simulink model "EPT"  (R2019b)
settings: Solver=FixedStepDiscrete  StartTime=0.0  StopTime=5  FixedStep=0.005  RelTol=1e-3  EnableMultiTasking=on
PreLoadFcn:
  | try, model_open; catch, disp('Error occurred while executing model pre-load callback: model_open.m'); disp('Please assure that the MATLAB working directory is set to the model directory before opening.'); end
InitFcn:
  | try, model_open; catch, end
undefined symbols (not defined in the file or in its folder): Bridge, GCM, H, ln, raptor_get_param_eval, raptor_get_safe_string, raptor_xcp_function
libraries: Raptor_lib x2810, simulink x374, hdlsllib x19
(part 35 of 45)

== system EPT/Foreground_TimeBase_5ms/E//W /BP-OBU_E//W/BP-OBU_E//W/BP-OBU_Warning//Fault_G3/BP-OBU_Warning_G3 ==
  Compare To Constant1 : simulink/Logic and Bit Operations/Compare To Constant  relop===  const=0  OutDataTypeStr=boolean
  Constant6 : Constant  Value=4
  Delay25 : Subsystem
  Delay26 : Subsystem
  Delay27 : Subsystem
  Delay28 : Subsystem
  Delay29 : Subsystem
  Latch26 : Subsystem
  Latch27 : Subsystem
  Latch28 : Subsystem
  Latch29 : Subsystem
  Logical Operator8 : Logic  Operator=OR  Inputs=7  AllPortsSameDT=off  OutDataTypeStr=boolean
  SOA : Subsystem
  raptor_adjustment82 : Raptor_lib/Data Storage/raptor_adjustment  paramName='Cdrive_Open'  nameSource=Parameter  initValue=0  dataType=boolean  storage=Calibration  calDispType=Number  calEnum={'False', 'True'}  calGain=1.0  calOffset=0.0  calMax=inf  calMin=-inf  calFormat='-1'  calUnit=''  calHelp=''  calAccess=1  calFunction=raptor_xcp_function(gcb)  calDispHeaders=off  calColHeaders={'Col1' 'Col2' 'Col3'}  calRowHeaders={'Row1' 'Row2' 'Row3'}
      settings: SourceProductName=Raptor
  raptor_adjustment83 : Raptor_lib/Data Storage/raptor_adjustment  paramName='Cchg_Open'  nameSource=Parameter  initValue=0  dataType=boolean  storage=Calibration  calDispType=Number  calEnum={'False', 'True'}  calGain=1.0  calOffset=0.0  calMax=inf  calMin=-inf  calFormat='-1'  calUnit=''  calHelp=''  calAccess=1  calFunction=raptor_xcp_function(gcb)  calDispHeaders=off  calColHeaders={'Col1' 'Col2' 'Col3'}  calRowHeaders={'Row1' 'Row2' 'Row3'}
      settings: SourceProductName=Raptor
  raptor_adjustment84 : Raptor_lib/Data Storage/raptor_adjustment  paramName='Caux_Open'  nameSource=Parameter  initValue=0  dataType=boolean  storage=Calibration  calDispType=Number  calEnum={'False', 'True'}  calGain=1.0  calOffset=0.0  calMax=inf  calMin=-inf  calFormat='-1'  calUnit=''  calHelp=''  calAccess=1  calFunction=raptor_xcp_function(gcb)  calDispHeaders=off  calColHeaders={'Col1' 'Col2' 'Col3'}  calRowHeaders={'Row1' 'Row2' 'Row3'}
      settings: SourceProductName=Raptor
  raptor_adjustment85 : Raptor_lib/Data Storage/raptor_adjustment  paramName='Csp_Open'  nameSource=Parameter  initValue=0  dataType=boolean  storage=Calibration  calDispType=Number  calEnum={'False', 'True'}  calGain=1.0  calOffset=0.0  calMax=inf  calMin=-inf  calFormat='-1'  calUnit=''  calHelp=''  calAccess=1  calFunction=raptor_xcp_function(gcb)  calDispHeaders=off  calColHeaders={'Col1' 'Col2' 'Col3'}  calRowHeaders={'Row1' 'Row2' 'Row3'}
      settings: SourceProductName=Raptor
  raptor_adjustment86 : Raptor_lib/Data Storage/raptor_adjustment  paramName='Fault_Cdrive_Open_1s_TimeCount'  nameSource=Parameter  initValue=200  dataType=double  storage=Calibration  calDispType=Number  calEnum={'False', 'True'}  calGain=1.0  calOffset=0.0  calMax=inf  calMin=-inf  calFormat='-1'  calUnit=''  calHelp=''  calAccess=1  calFunction=raptor_xcp_function(gcb)  calDispHeaders=off  calColHeaders={'Col1' 'Col2' 'Col3'}  calRowHeaders={'Row1' 'Row2' 'Row3'}
      settings: SourceProductName=Raptor
  raptor_adjustment87 : Raptor_lib/Data Storage/raptor_adjustment  paramName='Fault_Cchg_Open_1s_TimeCount'  nameSource=Parameter  initValue=200  dataType=double  storage=Calibration  calDispType=Number  calEnum={'False', 'True'}  calGain=1.0  calOffset=0.0  calMax=inf  calMin=-inf  calFormat='-1'  calUnit=''  calHelp=''  calAccess=1  calFunction=raptor_xcp_function(gcb)  calDispHeaders=off  calColHeaders={'Col1' 'Col2' 'Col3'}  calRowHeaders={'Row1' 'Row2' 'Row3'}
      settings: SourceProductName=Raptor
  raptor_adjustment88 : Raptor_lib/Data Storage/raptor_adjustment  paramName='Fault_Caux_Open_1s_TimeCount'  nameSource=Parameter  initValue=200  dataType=double  storage=Calibration  calDispType=Number  calEnum={'False', 'True'}  calGain=1.0  calOffset=0.0  calMax=inf  calMin=-inf  calFormat='-1'  calUnit=''  calHelp=''  calAccess=1  calFunction=raptor_xcp_function(gcb)  calDispHeaders=off  calColHeaders={'Col1' 'Col2' 'Col3'}  calRowHeaders={'Row1' 'Row2' 'Row3'}
      settings: SourceProductName=Raptor
  raptor_adjustment89 : Raptor_lib/Data Storage/raptor_adjustment  paramName='Fault_Csp_Open_1s_TimeCount'  nameSource=Parameter  initValue=200  dataType=double  storage=Calibration  calDispType=Number  calEnum={'False', 'True'}  calGain=1.0  calOffset=0.0  calMax=inf  calMin=-inf  calFormat='-1'  calUnit=''  calHelp=''  calAccess=1  calFunction=raptor_xcp_function(gcb)  calDispHeaders=off  calColHeaders={'Col1' 'Col2' 'Col3'}  calRowHeaders={'Row1' 'Row2' 'Row3'}
      settings: SourceProductName=Raptor
  raptor_data_def1 : Raptor_lib/Data Storage/raptor_data_def  dataName='Fault_SOA_OutOfRange'  initValue=0  dataType=boolean  storage=Calibration  calVisible=on  calType=Measurement  calDispType=Number  calEnum={'False', 'True'}  calGain=1.0  calOffset=0  calMin=-inf  calMax=inf  calFormat='-1'  calUnit=''  calHelp=''  calAccess=1  calFunction=raptor_xcp_function(gcb)  calDispHeaders=off  calColHeaders={'Col1' 'Col2' 'Col3'}  calRowHeaders={'Row1' 'Row2' 'Row3'}
      settings: SourceProductName=Raptor
  raptor_data_def10 : Raptor_lib/Data Storage/raptor_data_def  dataName='Warning_Cchg_Open'  initValue=0  dataType=boolean  storage=Calibration  calVisible=on  calType=Measurement  calDispType=Number  calEnum={'False', 'True'}  calGain=1.0  calOffset=0  calMin=-inf  calMax=inf  calFormat='-1'  calUnit=''  calHelp=''  calAccess=1  calFunction=raptor_xcp_function(gcb)  calDispHeaders=off  calColHeaders={'Col1' 'Col2' 'Col3'}  calRowHeaders={'Row1' 'Row2' 'Row3'}
      settings: SourceProductName=Raptor
  raptor_data_def11 : Raptor_lib/Data Storage/raptor_data_def  dataName='Warning_Caux_Open'  initValue=0  dataType=boolean  storage=Calibration  calVisible=on  calType=Measurement  calDispType=Number  calEnum={'False', 'True'}  calGain=1.0  calOffset=0  calMin=-inf  calMax=inf  calFormat='-1'  calUnit=''  calHelp=''  calAccess=1  calFunction=raptor_xcp_function(gcb)  calDispHeaders=off  calColHeaders={'Col1' 'Col2' 'Col3'}  calRowHeaders={'Row1' 'Row2' 'Row3'}
      settings: SourceProductName=Raptor
  raptor_data_def12 : Raptor_lib/Data Storage/raptor_data_def  dataName='Warning_Csp_Open'  initValue=0  dataType=boolean  storage=Calibration  calVisible=on  calType=Measurement  calDispType=Number  calEnum={'False', 'True'}  calGain=1.0  calOffset=0  calMin=-inf  calMax=inf  calFormat='-1'  calUnit=''  calHelp=''  calAccess=1  calFunction=raptor_xcp_function(gcb)  calDispHeaders=off  calColHeaders={'Col1' 'Col2' 'Col3'}  calRowHeaders={'Row1' 'Row2' 'Row3'}
      settings: SourceProductName=Raptor
  raptor_data_def2 : Raptor_lib/Data Storage/raptor_data_def  dataName='Warning_EndOfDischarge'  initValue=0  dataType=boolean  storage=Calibration  calVisible=on  calType=Measurement  calDispType=Number  calEnum={'False', 'True'}  calGain=1.0  calOffset=0  calMin=-inf  calMax=inf  calFormat='-1'  calUnit=''  calHelp=''  calAccess=1  calFunction=raptor_xcp_function(gcb)  calDispHeaders=off  calColHeaders={'Col1' 'Col2' 'Col3'}  calRowHeaders={'Row1' 'Row2' 'Row3'}
      settings: SourceProductName=Raptor
  raptor_data_def27 : Raptor_lib/Data Storage/raptor_data_def  dataName='Warning_EndOfCharge'  initValue=0  dataType=boolean  storage=Calibration  calVisible=on  calType=Measurement  calDispType=Number  calEnum={'False', 'True'}  calGain=1.0  calOffset=0  calMin=-inf  calMax=inf  calFormat='-1'  calUnit=''  calHelp=''  calAccess=1  calFunction=raptor_xcp_function(gcb)  calDispHeaders=off  calColHeaders={'Col1' 'Col2' 'Col3'}  calRowHeaders={'Row1' 'Row2' 'Row3'}
      settings: SourceProductName=Raptor
  raptor_data_def3 : Raptor_lib/Data Storage/raptor_data_def  dataName='Warning_SOA_OutOfRange'  initValue=0  dataType=boolean  storage=Calibration  calVisible=on  calType=Measurement  calDispType=Number  calEnum={'False', 'True'}  calGain=1.0  calOffset=0  calMin=-inf  calMax=inf  calFormat='-1'  calUnit=''  calHelp=''  calAccess=1  calFunction=raptor_xcp_function(gcb)  calDispHeaders=off  calColHeaders={'Col1' 'Col2' 'Col3'}  calRowHeaders={'Row1' 'Row2' 'Row3'}
      settings: SourceProductName=Raptor
  raptor_data_def4 : Raptor_lib/Data Storage/raptor_data_def  dataName='Fault_Cdrive_Open'  initValue=0  dataType=boolean  storage=Calibration  calVisible=on  calType=Measurement  calDispType=Number  calEnum={'False', 'True'}  calGain=1.0  calOffset=0  calMin=-inf  calMax=inf  calFormat='-1'  calUnit=''  calHelp=''  calAccess=1  calFunction=raptor_xcp_function(gcb)  calDispHeaders=off  calColHeaders={'Col1' 'Col2' 'Col3'}  calRowHeaders={'Row1' 'Row2' 'Row3'}
      settings: SourceProductName=Raptor
  raptor_data_def5 : Raptor_lib/Data Storage/raptor_data_def  dataName='Fault_Cchg_Open'  initValue=0  dataType=boolean  storage=Calibration  calVisible=on  calType=Measurement  calDispType=Number  calEnum={'False', 'True'}  calGain=1.0  calOffset=0  calMin=-inf  calMax=inf  calFormat='-1'  calUnit=''  calHelp=''  calAccess=1  calFunction=raptor_xcp_function(gcb)  calDispHeaders=off  calColHeaders={'Col1' 'Col2' 'Col3'}  calRowHeaders={'Row1' 'Row2' 'Row3'}
      settings: SourceProductName=Raptor
  raptor_data_def6 : Raptor_lib/Data Storage/raptor_data_def  dataName='Fault_Caux_Open'  initValue=0  dataType=boolean  storage=Calibration  calVisible=on  calType=Measurement  calDispType=Number  calEnum={'False', 'True'}  calGain=1.0  calOffset=0  calMin=-inf  calMax=inf  calFormat='-1'  calUnit=''  calHelp=''  calAccess=1  calFunction=raptor_xcp_function(gcb)  calDispHeaders=off  calColHeaders={'Col1' 'Col2' 'Col3'}  calRowHeaders={'Row1' 'Row2' 'Row3'}
      settings: SourceProductName=Raptor
  raptor_data_def7 : Raptor_lib/Data Storage/raptor_data_def  dataName='Fault_Csp_Open'  initValue=0  dataType=boolean  storage=Calibration  calVisible=on  calType=Measurement  calDispType=Number  calEnum={'False', 'True'}  calGain=1.0  calOffset=0  calMin=-inf  calMax=inf  calFormat='-1'  calUnit=''  calHelp=''  calAccess=1  calFunction=raptor_xcp_function(gcb)  calDispHeaders=off  calColHeaders={'Col1' 'Col2' 'Col3'}  calRowHeaders={'Row1' 'Row2' 'Row3'}
      settings: SourceProductName=Raptor
  raptor_data_def8 : Raptor_lib/Data Storage/raptor_data_def  dataName='HV_Off'  initValue=0  dataType=boolean  storage=Calibration  calVisible=on  calType=Measurement  calDispType=Number  calEnum={'False', 'True'}  calGain=1.0  calOffset=0  calMin=-inf  calMax=inf  calFormat='-1'  calUnit=''  calHelp=''  calAccess=1  calFunction=raptor_xcp_function(gcb)  calDispHeaders=off  calColHeaders={'Col1' 'Col2' 'Col3'}  calRowHeaders={'Row1' 'Row2' 'Row3'}
      settings: SourceProductName=Raptor
  raptor_data_def9 : Raptor_lib/Data Storage/raptor_data_def  dataName='Warning_Cdrive_Open'  initValue=0  dataType=boolean  storage=Calibration  calVisible=on  calType=Measurement  calDispType=Number  calEnum={'False', 'True'}  calGain=1.0  calOffset=0  calMin=-inf  calMax=inf  calFormat='-1'  calUnit=''  calHelp=''  calAccess=1  calFunction=raptor_xcp_function(gcb)  calDispHeaders=off  calColHeaders={'Col1' 'Col2' 'Col3'}  calRowHeaders={'Row1' 'Row2' 'Row3'}
      settings: SourceProductName=Raptor
  raptor_data_read : Raptor_lib/Data Storage/raptor_data_read  dataName='Warning_EndOfCharge'  dataShape=Scalar  idxSource=Input  idxRow=1  idxCol=1
      settings: SourceProductName=Raptor
  raptor_data_read1 : Raptor_lib/Data Storage/raptor_data_read  dataName='Warning_EndOfDischarge'  dataShape=Scalar  idxSource=Input  idxRow=1  idxCol=1
      settings: SourceProductName=Raptor
  raptor_data_read14 : Raptor_lib/Data Storage/raptor_data_read  dataName='Fault_Reset_Trigger'  dataShape=Scalar  idxSource=Input  idxRow=1  idxCol=1
      settings: SourceProductName=Raptor
  raptor_data_read3 : Raptor_lib/Data Storage/raptor_data_read  dataName='CMU_Ready'  dataShape=Scalar  idxSource=Input  idxRow=1  idxCol=1
      settings: SourceProductName=Raptor
  raptor_data_write10 : Raptor_lib/Data Storage/raptor_data_write  dataName='Warning_Cchg_Open'  dataShape=Scalar  idxSource=Input Port  idxRow=1  idxCol=1
      settings: SourceProductName=Raptor
  raptor_data_write11 : Raptor_lib/Data Storage/raptor_data_write  dataName='Warning_Csp_Open'  dataShape=Scalar  idxSource=Input Port  idxRow=1  idxCol=1
      settings: SourceProductName=Raptor
  raptor_data_write3 : Raptor_lib/Data Storage/raptor_data_write  dataName='Fault_Caux_Open'  dataShape=Scalar  idxSource=Input Port  idxRow=1  idxCol=1
      settings: SourceProductName=Raptor
  raptor_data_write4 : Raptor_lib/Data Storage/raptor_data_write  dataName='Fault_Cdrive_Open'  dataShape=Scalar  idxSource=Input Port  idxRow=1  idxCol=1
      settings: SourceProductName=Raptor
  raptor_data_write5 : Raptor_lib/Data Storage/raptor_data_write  dataName='Fault_Cchg_Open'  dataShape=Scalar  idxSource=Input Port  idxRow=1  idxCol=1
      settings: SourceProductName=Raptor
  raptor_data_write6 : Raptor_lib/Data Storage/raptor_data_write  dataName='Fault_Csp_Open'  dataShape=Scalar  idxSource=Input Port  idxRow=1  idxCol=1
      settings: SourceProductName=Raptor
  raptor_data_write7 : Raptor_lib/Data Storage/raptor_data_write  dataName='HV_Off'  dataShape=Scalar  idxSource=Input Port  idxRow=1  idxCol=1
      settings: SourceProductName=Raptor
  raptor_data_write8 : Raptor_lib/Data Storage/raptor_data_write  dataName='Warning_Caux_Open'  dataShape=Scalar  idxSource=Input Port  idxRow=1  idxCol=1
      settings: SourceProductName=Raptor
  raptor_data_write9 : Raptor_lib/Data Storage/raptor_data_write  dataName='Warning_Cdrive_Open'  dataShape=Scalar  idxSource=Input Port  idxRow=1  idxCol=1
      settings: SourceProductName=Raptor
  raptor_override : Raptor_lib/Data Storage/raptor_override  paramName='Cal_HV_Off'  nameSource=Parameter  measurement=None  calDispType=Number  calEnum={'False', 'True'}  calGain=1.0  calOffset=0.0  calMax=inf  calMin=-inf  calFormat='-1'  calUnit=''  calHelp=''  calAccess=1  calFunction=[raptor_xcp_function(gcb) '|' raptor_get_param_eval(gcb, 'paramName') '_Override']
      settings: SourceProductName=Raptor
  Warning_SOA_OutOfRange : Outport  VectorParamsAs1DForOutWhenUnconnected=off
  Warning_CMU_Status : Outport  Port=2  VectorParamsAs1DForOutWhenUnconnected=off
  Warning_Cdrive_Open : Outport  Port=3  VectorParamsAs1DForOutWhenUnconnected=off
  Warning_Cchg_Open : Outport  Port=4  VectorParamsAs1DForOutWhenUnconnected=off
  Warning_Caux_Open : Outport  Port=5  VectorParamsAs1DForOutWhenUnconnected=off
  Warning_Csp_Open : Outport  Port=6  VectorParamsAs1DForOutWhenUnconnected=off
  Fault_Cdrive_Open : Outport  Port=7  VectorParamsAs1DForOutWhenUnconnected=off
  Fault_Cchg_Open : Outport  Port=8  VectorParamsAs1DForOutWhenUnconnected=off
  Warning_Cdrive_Open3 : Outport  Port=9  VectorParamsAs1DForOutWhenUnconnected=off
  Fault_Csp_Open : Outport  Port=10  VectorParamsAs1DForOutWhenUnconnected=off
  wires:
  Latch28/1(Output) -> Warning_Cdrive_Open3/1, raptor_data_write3/1
  Delay27/1(Output) -> Latch27/1(Latch)
  Compare To Constant1/1 -> Delay25/1(Condition), Warning_CMU_Status/1
  raptor_adjustment82/1 -> Delay26/1(Condition), Logical Operator8/4, Warning_Cdrive_Open/1, raptor_data_write9/1
  raptor_data_read3/1 -> Compare To Constant1/1
  raptor_adjustment86/1 -> Delay26/2(TimeCount)
  Latch27/1(Output) -> Fault_Cchg_Open/1, raptor_data_write5/1
  Delay26/1(Output) -> Latch26/1(Latch)
  raptor_adjustment84/1 -> Delay28/1(Condition), Logical Operator8/6, Warning_Caux_Open/1, raptor_data_write8/1
  Logical Operator8/1 -> raptor_override/1
  raptor_adjustment89/1 -> Delay29/2(TimeCount)
  Latch29/1(Output) -> Fault_Csp_Open/1, raptor_data_write6/1
  raptor_adjustment85/1 -> Delay29/1(Condition), Logical Operator8/7, raptor_data_write11/1, Warning_Csp_Open/1
  raptor_adjustment87/1 -> Delay27/2(TimeCount)
  Latch26/1(Output) -> Fault_Cdrive_Open/1, raptor_data_write4/1
  Delay25/1(Output) -> Logical Operator8/3
  Constant6/1 -> Delay25/2(TimeCount)
  Delay29/1(Output) -> Latch29/1(Latch)
  Delay28/1(Output) -> Latch28/1(Latch)
  raptor_adjustment88/1 -> Delay28/2(TimeCount)
  raptor_adjustment83/1 -> Delay27/1(Condition), Logical Operator8/5, raptor_data_write10/1, Warning_Cchg_Open/1
  raptor_data_read14/1 -> Latch26/2(Reset), Latch27/2(Reset), Latch28/2(Reset), Latch29/2(Reset)
  raptor_data_read/1 -> Logical Operator8/1
  raptor_data_read1/1 -> Logical Operator8/2
  SOA/1(Out1) -> Warning_SOA_OutOfRange/1
  raptor_override/1 -> raptor_data_write7/1

== system EPT/Foreground_TimeBase_5ms/E//W /BP-OBU_E//W/BP-OBU_E//W/BP-OBU_Warning//Fault_G5/BP-OBU_Fault_G5 ==
  "MCU Work " : Inport
  Delay : Subsystem
  Delay1 : Subsystem
  Delay2 : Subsystem
  Delay3 : Subsystem
  Delay4 : Subsystem
  Delay5 : Subsystem
  Delay6 : Subsystem
  Error : Subsystem
  Error1 : Subsystem
  Error2 : Subsystem
  Error3 : Subsystem
  Error5 : Subsystem
  Error6 : Subsystem
  Error7 : Subsystem
  Logical Operator11 : Logic  AllPortsSameDT=off  OutDataTypeStr=boolean
  Logical Operator12 : Logic  AllPortsSameDT=off  OutDataTypeStr=boolean
  Logical Operator13 : Logic  AllPortsSameDT=off  OutDataTypeStr=boolean
  Relational Operator10 : RelationalOperator  Operator=<=  OutDataTypeStr=boolean  RndMeth=Simplest
  Relational Operator{7,9,12..14} (5 alike) : RelationalOperator  OutDataTypeStr=boolean  RndMeth=Simplest
  Relational Operator8 : RelationalOperator  Operator=<=  OutDataTypeStr=boolean  RndMeth=Simplest
  raptor_adjustment10 : Raptor_lib/Data Storage/raptor_adjustment  paramName='Fault__Sensor_Voltage_LowerLimit'  nameSource=Parameter  initValue=4  dataType=double  storage=Calibration  calDispType=Number  calEnum={'False', 'True'}  calGain=1.0  calOffset=0.0  calMax=inf  calMin=-inf  calFormat='-1'  calUnit=''  calHelp=''  calAccess=1  calFunction=raptor_xcp_function(gcb)  calDispHeaders=off  calColHeaders={'Col1' 'Col2' 'Col3'}  calRowHeaders={'Row1' 'Row2' 'Row3'}
      settings: SourceProductName=Raptor
  raptor_adjustment11 : Raptor_lib/Data Storage/raptor_adjustment  paramName='Fault_Sensor_Voltage_TimeCount'  nameSource=Parameter  initValue=20  dataType=double  storage=Calibration  calDispType=Number  calEnum={'False', 'True'}  calGain=1.0  calOffset=0.0  calMax=inf  calMin=-inf  calFormat='-1'  calUnit=''  calHelp=''  calAccess=1  calFunction=raptor_xcp_function(gcb)  calDispHeaders=off  calColHeaders={'Col1' 'Col2' 'Col3'}  calRowHeaders={'Row1' 'Row2' 'Row3'}
      settings: SourceProductName=Raptor
  raptor_adjustment12 : Raptor_lib/Data Storage/raptor_adjustment  paramName='Fault_Temperature_MCU_UpperLimit'  nameSource=Parameter  initValue=85  dataType=double  storage=Calibration  calDispType=Number  calEnum={'False', 'True'}  calGain=1.0  calOffset=0.0  calMax=inf  calMin=-inf  calFormat='-1'  calUnit=''  calHelp=''  calAccess=1  calFunction=raptor_xcp_function(gcb)  calDispHeaders=off  calColHeaders={'Col1' 'Col2' 'Col3'}  calRowHeaders={'Row1' 'Row2' 'Row3'}
      settings: SourceProductName=Raptor
  raptor_adjustment13 : Raptor_lib/Data Storage/raptor_adjustment  paramName='Fault_Temperature_Motor_UpperLimit'  nameSource=Parameter  initValue=135  dataType=double  storage=Calibration  calDispType=Number  calEnum={'False', 'True'}  calGain=1.0  calOffset=0.0  calMax=inf  calMin=-inf  calFormat='-1'  calUnit=''  calHelp=''  calAccess=1  calFunction=raptor_xcp_function(gcb)  calDispHeaders=off  calColHeaders={'Col1' 'Col2' 'Col3'}  calRowHeaders={'Row1' 'Row2' 'Row3'}
      settings: SourceProductName=Raptor
  raptor_adjustment14 : Raptor_lib/Data Storage/raptor_adjustment  paramName='Fault_Motor_RPM_UpperLimit'  nameSource=Parameter  initValue=6500  dataType=double  storage=Calibration  calDispType=Number  calEnum={'False', 'True'}  calGain=1.0  calOffset=0.0  calMax=inf  calMin=-inf  calFormat='-1'  calUnit=''  calHelp=''  calAccess=1  calFunction=raptor_xcp_function(gcb)  calDispHeaders=off  calColHeaders={'Col1' 'Col2' 'Col3'}  calRowHeaders={'Row1' 'Row2' 'Row3'}
      settings: SourceProductName=Raptor
  raptor_adjustment15 : Raptor_lib/Data Storage/raptor_adjustment  paramName='Fault_Motor_RPM_TimeCount'  nameSource=Parameter  initValue=20  dataType=double  storage=Calibration  calDispType=Number  calEnum={'False', 'True'}  calGain=1.0  calOffset=0.0  calMax=inf  calMin=-inf  calFormat='-1'  calUnit=''  calHelp=''  calAccess=1  calFunction=raptor_xcp_function(gcb)  calDispHeaders=off  calColHeaders={'Col1' 'Col2' 'Col3'}  calRowHeaders={'Row1' 'Row2' 'Row3'}
      settings: SourceProductName=Raptor
  raptor_adjustment16 : Raptor_lib/Data Storage/raptor_adjustment  paramName='Fault_Temperature_Motor_TimeCount'  nameSource=Parameter  initValue=20  dataType=double  storage=Calibration  calDispType=Number  calEnum={'False', 'True'}  calGain=1.0  calOffset=0.0  calMax=inf  calMin=-inf  calFormat='-1'  calUnit=''  calHelp=''  calAccess=1  calFunction=raptor_xcp_function(gcb)  calDispHeaders=off  calColHeaders={'Col1' 'Col2' 'Col3'}  calRowHeaders={'Row1' 'Row2' 'Row3'}
      settings: SourceProductName=Raptor
  raptor_adjustment17 : Raptor_lib/Data Storage/raptor_adjustment  paramName='Fault_Temperature_MCU_TimeCount'  nameSource=Parameter  initValue=20  dataType=double  storage=Calibration  calDispType=Number  calEnum={'False', 'True'}  calGain=1.0  calOffset=0.0  calMax=inf  calMin=-inf  calFormat='-1'  calUnit=''  calHelp=''  calAccess=1  calFunction=raptor_xcp_function(gcb)  calDispHeaders=off  calColHeaders={'Col1' 'Col2' 'Col3'}  calRowHeaders={'Row1' 'Row2' 'Row3'}
      settings: SourceProductName=Raptor
  raptor_adjustment4 : Raptor_lib/Data Storage/raptor_adjustment  paramName='Fault_12VBattery_Voltage_TimeCount'  nameSource=Parameter  initValue=20  dataType=double  storage=Calibration  calDispType=Number  calEnum={'False', 'True'}  calGain=1.0  calOffset=0.0  calMax=inf  calMin=-inf  calFormat='-1'  calUnit=''  calHelp=''  calAccess=1  calFunction=raptor_xcp_function(gcb)  calDispHeaders=off  calColHeaders={'Col1' 'Col2' 'Col3'}  calRowHeaders={'Row1' 'Row2' 'Row3'}
      settings: SourceProductName=Raptor
  raptor_adjustment7 : Raptor_lib/Data Storage/raptor_adjustment  paramName='Fault_Battery_Voltage_UpperLimit'  nameSource=Parameter  initValue=15  dataType=double  storage=Calibration  calDispType=Number  calEnum={'False', 'True'}  calGain=1.0  calOffset=0.0  calMax=inf  calMin=-inf  calFormat='-1'  calUnit=''  calHelp=''  calAccess=1  calFunction=raptor_xcp_function(gcb)  calDispHeaders=off  calColHeaders={'Col1' 'Col2' 'Col3'}  calRowHeaders={'Row1' 'Row2' 'Row3'}
      settings: SourceProductName=Raptor
  raptor_adjustment8 : Raptor_lib/Data Storage/raptor_adjustment  paramName='Fault__Battery_Voltage_LowerLimit'  nameSource=Parameter  initValue=10  dataType=double  storage=Calibration  calDispType=Number  calEnum={'False', 'True'}  calGain=1.0  calOffset=0.0  calMax=inf  calMin=-inf  calFormat='-1'  calUnit=''  calHelp=''  calAccess=1  calFunction=raptor_xcp_function(gcb)  calDispHeaders=off  calColHeaders={'Col1' 'Col2' 'Col3'}  calRowHeaders={'Row1' 'Row2' 'Row3'}
      settings: SourceProductName=Raptor
  raptor_adjustment9 : Raptor_lib/Data Storage/raptor_adjustment  paramName='Fault_Sensor_Voltage_UpperLimit'  nameSource=Parameter  initValue=6  dataType=double  storage=Calibration  calDispType=Number  calEnum={'False', 'True'}  calGain=1.0  calOffset=0.0  calMax=inf  calMin=-inf  calFormat='-1'  calUnit=''  calHelp=''  calAccess=1  calFunction=raptor_xcp_function(gcb)  calDispHeaders=off  calColHeaders={'Col1' 'Col2' 'Col3'}  calRowHeaders={'Row1' 'Row2' 'Row3'}
      settings: SourceProductName=Raptor
  raptor_data_def11 : Raptor_lib/Data Storage/raptor_data_def  dataName='Fault_12V_Battery_Voltage_Low'  initValue=0  dataType=boolean  storage=Volatile (RAM)  calVisible=on  calType=Measurement  calDispType=Number  calEnum={'False', 'True'}  calGain=1.0  calOffset=0  calMin=-inf  calMax=inf  calFormat='-1'  calUnit=''  calHelp=''  calAccess=1  calFunction=raptor_xcp_function(gcb)  calDispHeaders=off  calColHeaders={'Col1' 'Col2' 'Col3'}  calRowHeaders={'Row1' 'Row2' 'Row3'}
      settings: SourceProductName=Raptor
  raptor_data_def12 : Raptor_lib/Data Storage/raptor_data_def  dataName='Fault_Sensor_Voltage_High'  initValue=0  dataType=boolean  storage=Volatile (RAM)  calVisible=on  calType=Measurement  calDispType=Number  calEnum={'False', 'True'}  calGain=1.0  calOffset=0  calMin=-inf  calMax=inf  calFormat='-1'  calUnit=''  calHelp=''  calAccess=1  calFunction=raptor_xcp_function(gcb)  calDispHeaders=off  calColHeaders={'Col1' 'Col2' 'Col3'}  calRowHeaders={'Row1' 'Row2' 'Row3'}
      settings: SourceProductName=Raptor
  raptor_data_def13 : Raptor_lib/Data Storage/raptor_data_def  dataName='Fault_Sensor_Voltage_Low'  initValue=0  dataType=boolean  storage=Volatile (RAM)  calVisible=on  calType=Measurement  calDispType=Number  calEnum={'False', 'True'}  calGain=1.0  calOffset=0  calMin=-inf  calMax=inf  calFormat='-1'  calUnit=''  calHelp=''  calAccess=1  calFunction=raptor_xcp_function(gcb)  calDispHeaders=off  calColHeaders={'Col1' 'Col2' 'Col3'}  calRowHeaders={'Row1' 'Row2' 'Row3'}
      settings: SourceProductName=Raptor
  raptor_data_def15 : Raptor_lib/Data Storage/raptor_data_def  dataName='Fault_Temperature_MCU_High'  initValue=0  dataType=boolean  storage=Volatile (RAM)  calVisible=on  calType=Measurement  calDispType=Number  calEnum={'False', 'True'}  calGain=1.0  calOffset=0  calMin=-inf  calMax=inf  calFormat='-1'  calUnit=''  calHelp=''  calAccess=1  calFunction=raptor_xcp_function(gcb)  calDispHeaders=off  calColHeaders={'Col1' 'Col2' 'Col3'}  calRowHeaders={'Row1' 'Row2' 'Row3'}
      settings: SourceProductName=Raptor
  raptor_data_def16 : Raptor_lib/Data Storage/raptor_data_def  dataName='Fault_Temperature_Motor_High'  initValue=0  dataType=boolean  storage=Volatile (RAM)  calVisible=on  calType=Measurement  calDispType=Number  calEnum={'False', 'True'}  calGain=1.0  calOffset=0  calMin=-inf  calMax=inf  calFormat='-1'  calUnit=''  calHelp=''  calAccess=1  calFunction=raptor_xcp_function(gcb)  calDispHeaders=off  calColHeaders={'Col1' 'Col2' 'Col3'}  calRowHeaders={'Row1' 'Row2' 'Row3'}
      settings: SourceProductName=Raptor
  raptor_data_def18 : Raptor_lib/Data Storage/raptor_data_def  dataName='Fault_Motor_RPM_High'  initValue=0  dataType=boolean  storage=Volatile (RAM)  calVisible=on  calType=Measurement  calDispType=Number  calEnum={'False', 'True'}  calGain=1.0  calOffset=0  calMin=-inf  calMax=inf  calFormat='-1'  calUnit=''  calHelp=''  calAccess=1  calFunction=raptor_xcp_function(gcb)  calDispHeaders=off  calColHeaders={'Col1' 'Col2' 'Col3'}  calRowHeaders={'Row1' 'Row2' 'Row3'}
      settings: SourceProductName=Raptor
  raptor_data_def9 : Raptor_lib/Data Storage/raptor_data_def  dataName='Fault_12V_Battery_Voltage_High'  initValue=0  dataType=boolean  storage=Volatile (RAM)  calVisible=on  calType=Measurement  calDispType=Number  calEnum={'False', 'True'}  calGain=1.0  calOffset=0  calMin=-inf  calMax=inf  calFormat='-1'  calUnit=''  calHelp=''  calAccess=1  calFunction=raptor_xcp_function(gcb)  calDispHeaders=off  calColHeaders={'Col1' 'Col2' 'Col3'}  calRowHeaders={'Row1' 'Row2' 'Row3'}
      settings: SourceProductName=Raptor
  raptor_data_read13 : Raptor_lib/Data Storage/raptor_data_read  dataName='Sensor_5V_Volt'  dataShape=Scalar  idxSource=Input  idxRow=1  idxCol=1
      settings: SourceProductName=Raptor
  raptor_data_read14 : Raptor_lib/Data Storage/raptor_data_read  dataName='Fault_Reset_Trigger'  dataShape=Scalar  idxSource=Input  idxRow=1  idxCol=1
      settings: SourceProductName=Raptor
  raptor_data_read4 : Raptor_lib/Data Storage/raptor_data_read  dataName='Read_Controller_Temp'  dataShape=Scalar  idxSource=Input  idxRow=1  idxCol=1
      settings: SourceProductName=Raptor
  raptor_data_read5 : Raptor_lib/Data Storage/raptor_data_read  dataName='Read_Motor_Temp'  dataShape=Scalar  idxSource=Input  idxRow=1  idxCol=1
      settings: SourceProductName=Raptor
  raptor_data_read6 : Raptor_lib/Data Storage/raptor_data_read  dataName='Read_Motor_Speed'  dataShape=Scalar  idxSource=Input  idxRow=1  idxCol=1
      settings: SourceProductName=Raptor
  raptor_data_read7 : Raptor_lib/Data Storage/raptor_data_read  dataName='I2V_Battery_Volt'  dataShape=Scalar  idxSource=Input  idxRow=1  idxCol=1
      settings: SourceProductName=Raptor
  raptor_data_write10 : Raptor_lib/Data Storage/raptor_data_write  dataName='Fault_Sensor_Voltage_High'  dataShape=Scalar  idxSource=Input Port  idxRow=1  idxCol=1
      settings: SourceProductName=Raptor
  raptor_data_write11 : Raptor_lib/Data Storage/raptor_data_write  dataName='Fault_12V_Battery_Voltage_High'  dataShape=Scalar  idxSource=Input Port  idxRow=1  idxCol=1
      settings: SourceProductName=Raptor
  raptor_data_write12 : Raptor_lib/Data Storage/raptor_data_write  dataName='Fault_12V_Battery_Voltage_Low'  dataShape=Scalar  idxSource=Input Port  idxRow=1  idxCol=1
      settings: SourceProductName=Raptor
  raptor_data_write13 : Raptor_lib/Data Storage/raptor_data_write  dataName='Fault_Sensor_Voltage_Low'  dataShape=Scalar  idxSource=Input Port  idxRow=1  idxCol=1
      settings: SourceProductName=Raptor
  raptor_data_write15 : Raptor_lib/Data Storage/raptor_data_write  dataName='Fault_Temperature_MCU_High'  dataShape=Scalar  idxSource=Input Port  idxRow=1  idxCol=1
      settings: SourceProductName=Raptor
  raptor_data_write16 : Raptor_lib/Data Storage/raptor_data_write  dataName='Fault_Temperature_Motor_High'  dataShape=Scalar  idxSource=Input Port  idxRow=1  idxCol=1
      settings: SourceProductName=Raptor
  raptor_data_write18 : Raptor_lib/Data Storage/raptor_data_write  dataName='Fault_Motor_RPM_High'  dataShape=Scalar  idxSource=Input Port  idxRow=1  idxCol=1
      settings: SourceProductName=Raptor
  wires:
  Delay2/1(Output) -> Error2/1(" Condition")
  raptor_data_read13/1 -> Relational Operator10/1, Relational Operator9/1
  raptor_adjustment15/1 -> Delay6/2(TimeCount)
  raptor_data_read14/1 -> Error7/2(" Reset"), Error6/2(" Reset"), Error5/2(" Reset"), Error3/2(" Reset"), Error2/2(" Reset"), Error1/2(" Reset"), Error/2(" Reset")
  raptor_data_read7/1 -> Relational Operator7/1, Relational Operator8/1
  "MCU Work "/1 -> Logical Operator13/1, Logical Operator12/1, Logical Operator11/1
  Logical Operator12/1 -> Delay5/1(Condition)
  Logical Operator11/1 -> Delay4/1(Condition)
  raptor_adjustment17/1 -> Delay4/2(TimeCount)
  Relational Operator9/1 -> Delay2/1(Condition)
  Relational Operator13/1 -> Logical Operator12/2
  Relational Operator10/1 -> Delay3/1(Condition)
  Error5/1(Error) -> raptor_data_write15/1
  raptor_adjustment4/1 -> Delay1/2(TimeCount), Delay/2(TimeCount)
  raptor_adjustment10/1 -> Relational Operator10/2
  raptor_adjustment12/1 -> Relational Operator12/2
  raptor_data_read4/1 -> Relational Operator12/1
  raptor_adjustment7/1 -> Relational Operator7/2
  Delay/1(Output) -> Error/1(" Condition")
  raptor_data_read5/1 -> Relational Operator13/1
  raptor_adjustment8/1 -> Relational Operator8/2
  raptor_adjustment14/1 -> Relational Operator14/2
  Error2/1(Error) -> raptor_data_write10/1
  raptor_adjustment9/1 -> Relational Operator9/2
  raptor_adjustment13/1 -> Relational Operator13/2
  Error1/1(Error) -> raptor_data_write12/1
  Relational Operator14/1 -> Logical Operator13/2
  Error3/1(Error) -> raptor_data_write13/1
  raptor_adjustment11/1 -> Delay2/2(TimeCount), Delay3/2(TimeCount)
  Relational Operator12/1 -> Logical Operator11/2
  Relational Operator7/1 -> Delay/1(Condition)
  Relational Operator8/1 -> Delay1/1(Condition)
  Logical Operator13/1 -> Delay6/1(Condition)
  Delay6/1(Output) -> Error7/1(" Condition")
  Delay3/1(Output) -> Error3/1(" Condition")
  raptor_adjustment16/1 -> Delay5/2(TimeCount)
  Delay1/1(Output) -> Error1/1(" Condition")
  Delay4/1(Output) -> Error5/1(" Condition")
  Delay5/1(Output) -> Error6/1(" Condition")
  Error/1(Error) -> raptor_data_write11/1
  raptor_data_read6/1 -> Relational Operator14/1
  Error7/1(Error) -> raptor_data_write18/1
  Error6/1(Error) -> raptor_data_write16/1

== system EPT/Foreground_TimeBase_5ms/E//W /BP-OBU_E//W/BP-OBU_E//W/BP-OBU_Warning//Fault_G5/BP-OBU_Warning_G5 ==
  "MCU Work " : Inport
  Logical Operator8 : Logic  AllPortsSameDT=off  OutDataTypeStr=boolean
  Logical Operator9 : Logic  AllPortsSameDT=off  OutDataTypeStr=boolean
  Relational Operator{,2,5..6} (4 alike) : RelationalOperator  OutDataTypeStr=boolean  RndMeth=Simplest
  Relational Operator1 : RelationalOperator  Operator=<=  OutDataTypeStr=boolean  RndMeth=Simplest
  Relational Operator3 : RelationalOperator  Operator=<=  OutDataTypeStr=boolean  RndMeth=Simplest
  raptor_adjustment : Raptor_lib/Data Storage/raptor_adjustment  paramName='Warning_12VBattery_Voltage_UpperLimit'  nameSource=Parameter  initValue=13.8  dataType=double  storage=Calibration  calDispType=Number  calEnum={'False', 'True'}  calGain=1.0  calOffset=0.0  calMax=inf  calMin=-inf  calFormat='-1'  calUnit=''  calHelp=''  calAccess=1  calFunction=raptor_xcp_function(gcb)  calDispHeaders=off  calColHeaders={'Col1' 'Col2' 'Col3'}  calRowHeaders={'Row1' 'Row2' 'Row3'}
      settings: SourceProductName=Raptor
  raptor_adjustment1 : Raptor_lib/Data Storage/raptor_adjustment  paramName='Warning_12VBattery_Voltage_LowerLimit'  nameSource=Parameter  initValue=11  dataType=double  storage=Calibration  calDispType=Number  calEnum={'False', 'True'}  calGain=1.0  calOffset=0.0  calMax=inf  calMin=-inf  calFormat='-1'  calUnit=''  calHelp=''  calAccess=1  calFunction=raptor_xcp_function(gcb)  calDispHeaders=off  calColHeaders={'Col1' 'Col2' 'Col3'}  calRowHeaders={'Row1' 'Row2' 'Row3'}
      settings: SourceProductName=Raptor
  raptor_adjustment2 : Raptor_lib/Data Storage/raptor_adjustment  paramName='Warning_Sensor_Voltage_UpperLimit'  nameSource=Parameter  initValue=5.5  dataType=double  storage=Calibration  calDispType=Number  calEnum={'False', 'True'}  calGain=1.0  calOffset=0.0  calMax=inf  calMin=-inf  calFormat='-1'  calUnit=''  calHelp=''  calAccess=1  calFunction=raptor_xcp_function(gcb)  calDispHeaders=off  calColHeaders={'Col1' 'Col2' 'Col3'}  calRowHeaders={'Row1' 'Row2' 'Row3'}
      settings: SourceProductName=Raptor
  raptor_adjustment3 : Raptor_lib/Data Storage/raptor_adjustment  paramName='Warning_Sensor_Voltage_LowerLimit'  nameSource=Parameter  initValue=4.5  dataType=double  storage=Calibration  calDispType=Number  calEnum={'False', 'True'}  calGain=1.0  calOffset=0.0  calMax=inf  calMin=-inf  calFormat='-1'  calUnit=''  calHelp=''  calAccess=1  calFunction=raptor_xcp_function(gcb)  calDispHeaders=off  calColHeaders={'Col1' 'Col2' 'Col3'}  calRowHeaders={'Row1' 'Row2' 'Row3'}
      settings: SourceProductName=Raptor
  raptor_adjustment5 : Raptor_lib/Data Storage/raptor_adjustment  paramName='Warning_Temperature_MCU_UpperLimit'  nameSource=Parameter  initValue=70  dataType=double  storage=Calibration  calDispType=Number  calEnum={'False', 'True'}  calGain=1.0  calOffset=0.0  calMax=inf  calMin=-inf  calFormat='-1'  calUnit=''  calHelp=''  calAccess=1  calFunction=raptor_xcp_function(gcb)  calDispHeaders=off  calColHeaders={'Col1' 'Col2' 'Col3'}  calRowHeaders={'Row1' 'Row2' 'Row3'}
      settings: SourceProductName=Raptor
  raptor_adjustment6 : Raptor_lib/Data Storage/raptor_adjustment  paramName='Warning_Temperature_Motor_UpperLimit'  nameSource=Parameter  initValue=100  dataType=double  storage=Calibration  calDispType=Number  calEnum={'False', 'True'}  calGain=1.0  calOffset=0.0  calMax=inf  calMin=-inf  calFormat='-1'  calUnit=''  calHelp=''  calAccess=1  calFunction=raptor_xcp_function(gcb)  calDispHeaders=off  calColHeaders={'Col1' 'Col2' 'Col3'}  calRowHeaders={'Row1' 'Row2' 'Row3'}
      settings: SourceProductName=Raptor
  raptor_data_def2 : Raptor_lib/Data Storage/raptor_data_def  dataName='Warning_12V_Battery_Voltage_High'  initValue=0  dataType=boolean  storage=Volatile (RAM)  calVisible=on  calType=Measurement  calDispType=Number  calEnum={'False', 'True'}  calGain=1.0  calOffset=0  calMin=-inf  calMax=inf  calFormat='-1'  calUnit=''  calHelp=''  calAccess=1  calFunction=raptor_xcp_function(gcb)  calDispHeaders=off  calColHeaders={'Col1' 'Col2' 'Col3'}  calRowHeaders={'Row1' 'Row2' 'Row3'}
      settings: SourceProductName=Raptor
  raptor_data_def3 : Raptor_lib/Data Storage/raptor_data_def  dataName='Warning_12V_Battery_Voltage_Low'  initValue=0  dataType=boolean  storage=Volatile (RAM)  calVisible=on  calType=Measurement  calDispType=Number  calEnum={'False', 'True'}  calGain=1.0  calOffset=0  calMin=-inf  calMax=inf  calFormat='-1'  calUnit=''  calHelp=''  calAccess=1  calFunction=raptor_xcp_function(gcb)  calDispHeaders=off  calColHeaders={'Col1' 'Col2' 'Col3'}  calRowHeaders={'Row1' 'Row2' 'Row3'}
      settings: SourceProductName=Raptor
  raptor_data_def4 : Raptor_lib/Data Storage/raptor_data_def  dataName='Warning_Sensor_Voltage_High'  initValue=0  dataType=boolean  storage=Volatile (RAM)  calVisible=on  calType=Measurement  calDispType=Number  calEnum={'False', 'True'}  calGain=1.0  calOffset=0  calMin=-inf  calMax=inf  calFormat='-1'  calUnit=''  calHelp=''  calAccess=1  calFunction=raptor_xcp_function(gcb)  calDispHeaders=off  calColHeaders={'Col1' 'Col2' 'Col3'}  calRowHeaders={'Row1' 'Row2' 'Row3'}
      settings: SourceProductName=Raptor
  raptor_data_def5 : Raptor_lib/Data Storage/raptor_data_def  dataName='Warning_Sensor_Voltage_Low'  initValue=0  dataType=boolean  storage=Volatile (RAM)  calVisible=on  calType=Measurement  calDispType=Number  calEnum={'False', 'True'}  calGain=1.0  calOffset=0  calMin=-inf  calMax=inf  calFormat='-1'  calUnit=''  calHelp=''  calAccess=1  calFunction=raptor_xcp_function(gcb)  calDispHeaders=off  calColHeaders={'Col1' 'Col2' 'Col3'}  calRowHeaders={'Row1' 'Row2' 'Row3'}
      settings: SourceProductName=Raptor
  raptor_data_def7 : Raptor_lib/Data Storage/raptor_data_def  dataName='Warning_Temperature_MCU_High'  initValue=0  dataType=boolean  storage=Volatile (RAM)  calVisible=on  calType=Measurement  calDispType=Number  calEnum={'False', 'True'}  calGain=1.0  calOffset=0  calMin=-inf  calMax=inf  calFormat='-1'  calUnit=''  calHelp=''  calAccess=1  calFunction=raptor_xcp_function(gcb)  calDispHeaders=off  calColHeaders={'Col1' 'Col2' 'Col3'}  calRowHeaders={'Row1' 'Row2' 'Row3'}
      settings: SourceProductName=Raptor
  raptor_data_def8 : Raptor_lib/Data Storage/raptor_data_def  dataName='Warning_Temperature_Motor_High'  initValue=0  dataType=boolean  storage=Volatile (RAM)  calVisible=on  calType=Measurement  calDispType=Number  calEnum={'False', 'True'}  calGain=1.0  calOffset=0  calMin=-inf  calMax=inf  calFormat='-1'  calUnit=''  calHelp=''  calAccess=1  calFunction=raptor_xcp_function(gcb)  calDispHeaders=off  calColHeaders={'Col1' 'Col2' 'Col3'}  calRowHeaders={'Row1' 'Row2' 'Row3'}
      settings: SourceProductName=Raptor
  raptor_data_read1 : Raptor_lib/Data Storage/raptor_data_read  dataName='Read_Controller_Temp'  dataShape=Scalar  idxSource=Input  idxRow=1  idxCol=1
      settings: SourceProductName=Raptor
  raptor_data_read11 : Raptor_lib/Data Storage/raptor_data_read  dataName='I2V_Battery_Volt'  dataShape=Scalar  idxSource=Input  idxRow=1  idxCol=1
      settings: SourceProductName=Raptor
  raptor_data_read12 : Raptor_lib/Data Storage/raptor_data_read  dataName='Sensor_5V_Volt'  dataShape=Scalar  idxSource=Input  idxRow=1  idxCol=1
      settings: SourceProductName=Raptor
  raptor_data_read2 : Raptor_lib/Data Storage/raptor_data_read  dataName='Read_Motor_Temp'  dataShape=Scalar  idxSource=Input  idxRow=1  idxCol=1
      settings: SourceProductName=Raptor
  raptor_data_write1 : Raptor_lib/Data Storage/raptor_data_write  dataName='Warning_Sensor_Voltage_High'  dataShape=Scalar  idxSource=Input Port  idxRow=1  idxCol=1
      settings: SourceProductName=Raptor
  raptor_data_write2 : Raptor_lib/Data Storage/raptor_data_write  dataName='Warning_12V_Battery_Voltage_High'  dataShape=Scalar  idxSource=Input Port  idxRow=1  idxCol=1
      settings: SourceProductName=Raptor
  raptor_data_write3 : Raptor_lib/Data Storage/raptor_data_write  dataName='Warning_12V_Battery_Voltage_Low'  dataShape=Scalar  idxSource=Input Port  idxRow=1  idxCol=1
      settings: SourceProductName=Raptor
  raptor_data_write4 : Raptor_lib/Data Storage/raptor_data_write  dataName='Warning_Sensor_Voltage_Low'  dataShape=Scalar  idxSource=Input Port  idxRow=1  idxCol=1
      settings: SourceProductName=Raptor
  raptor_data_write6 : Raptor_lib/Data Storage/raptor_data_write  dataName='Warning_Temperature_MCU_High'  dataShape=Scalar  idxSource=Input Port  idxRow=1  idxCol=1
      settings: SourceProductName=Raptor
  raptor_data_write7 : Raptor_lib/Data Storage/raptor_data_write  dataName='Warning_Temperature_Motor_High'  dataShape=Scalar  idxSource=Input Port  idxRow=1  idxCol=1
      settings: SourceProductName=Raptor
  wires:
  raptor_adjustment1/1 -> Relational Operator1/2
  raptor_adjustment/1 -> Relational Operator/2
  raptor_adjustment3/1 -> Relational Operator3/2
  "MCU Work "/1 -> Logical Operator9/1, Logical Operator8/1
  raptor_data_read11/1 -> Relational Operator/1, Relational Operator1/1
  Relational Operator2/1 -> raptor_data_write1/1
  raptor_adjustment5/1 -> Relational Operator5/2
  raptor_adjustment2/1 -> Relational Operator2/2
  raptor_data_read1/1 -> Relational Operator5/1
  Relational Operator5/1 -> Logical Operator8/2
  raptor_data_read2/1 -> Relational Operator6/1
  Relational Operator6/1 -> Logical Operator9/2
  Relational Operator1/1 -> raptor_data_write3/1
  Logical Operator9/1 -> raptor_data_write7/1
  Relational Operator/1 -> raptor_data_write2/1
  Relational Operator3/1 -> raptor_data_write4/1
  Logical Operator8/1 -> raptor_data_write6/1
  raptor_data_read12/1 -> Relational Operator2/1, Relational Operator3/1
  raptor_adjustment6/1 -> Relational Operator6/2

== system EPT/Foreground_TimeBase_5ms/E//W /BP-OBU_E//W/BP-OBU_E//W/BP-OBU_Warning//Fault_G5/Delay37 ==
  Condition : Inport
  TimeCount : Inport  Port=2
  Constant10 : Constant
  Constant11 : Constant  Value=0
  Constant8 : Constant  Value=0
  CycleTrigger : Subsystem
  Switch2 : Switch  Threshold=1
  Switch3 : Switch  Threshold=1
  Unit Delay1 : UnitDelay  SampleTime=-1  HasFrameUpgradeWarning=on
  Unit Delay2 : UnitDelay  SampleTime=-1  HasFrameUpgradeWarning=on
  Output : Outport  VectorParamsAs1DForOutWhenUnconnected=off
  wires:
  Unit Delay1/1 -> Output/1
  Switch2/1 -> Unit Delay2/1
  Unit Delay2/1 -> Switch3/1
  Constant11/1 -> Switch3/3
  Switch3/1 -> CycleTrigger/1(In1)
  Constant10/1 -> Switch2/3
  Constant8/1 -> Switch2/1
  CycleTrigger/1(Trigger) -> Unit Delay1/1, Switch2/2
  Condition/1 -> Switch3/2
  TimeCount/1 -> CycleTrigger/2(In2)

== system EPT/Foreground_TimeBase_5ms/E//W /BP-OBU_E//W/BP-OBU_E//W/BP-OBU_Warning//Fault_G5/Delay38 ==
  Condition : Inport
  TimeCount : Inport  Port=2
  Constant10 : Constant
  Constant11 : Constant  Value=0
  Constant8 : Constant  Value=0
  CycleTrigger : Subsystem
  Switch2 : Switch  Threshold=1
  Switch3 : Switch  Threshold=1
  Unit Delay1 : UnitDelay  SampleTime=-1  HasFrameUpgradeWarning=on
  Unit Delay2 : UnitDelay  SampleTime=-1  HasFrameUpgradeWarning=on
  Output : Outport  VectorParamsAs1DForOutWhenUnconnected=off
  wires:
  TimeCount/1 -> CycleTrigger/2(In2)
  Condition/1 -> Switch3/2
  CycleTrigger/1(Trigger) -> Switch2/2, Unit Delay1/1
  Constant8/1 -> Switch2/1
  Constant10/1 -> Switch2/3
  Switch3/1 -> CycleTrigger/1(In1)
  Constant11/1 -> Switch3/3
  Unit Delay2/1 -> Switch3/1
  Switch2/1 -> Unit Delay2/1
  Unit Delay1/1 -> Output/1

== system EPT/Foreground_TimeBase_5ms/E//W /BP-OBU_E//W/BP-OBU_E//W/BP-OBU_Warning//Fault_G5/Delay39 ==
  Condition : Inport
  TimeCount : Inport  Port=2
  Constant10 : Constant
  Constant11 : Constant  Value=0
  Constant8 : Constant  Value=0
  CycleTrigger : Subsystem
  Switch2 : Switch  Threshold=1
  Switch3 : Switch  Threshold=1
  Unit Delay1 : UnitDelay  SampleTime=-1  HasFrameUpgradeWarning=on
  Unit Delay2 : UnitDelay  SampleTime=-1  HasFrameUpgradeWarning=on
  Output : Outport  VectorParamsAs1DForOutWhenUnconnected=off
  wires:
  Unit Delay1/1 -> Output/1
  Switch2/1 -> Unit Delay2/1
  Unit Delay2/1 -> Switch3/1
  Constant11/1 -> Switch3/3
  Switch3/1 -> CycleTrigger/1(In1)
  Constant10/1 -> Switch2/3
  Constant8/1 -> Switch2/1
  CycleTrigger/1(Trigger) -> Unit Delay1/1, Switch2/2
  Condition/1 -> Switch3/2
  TimeCount/1 -> CycleTrigger/2(In2)

== system EPT/Foreground_TimeBase_5ms/E//W /BP-OBU_E//W/BP-OBU_E//W/BP-OBU_Warning//Fault_G5/Delay40 ==
  Condition : Inport
  TimeCount : Inport  Port=2
  Constant10 : Constant
  Constant11 : Constant  Value=0
  Constant8 : Constant  Value=0
  CycleTrigger : Subsystem
  Switch2 : Switch  Threshold=1
  Switch3 : Switch  Threshold=1
  Unit Delay1 : UnitDelay  SampleTime=-1  HasFrameUpgradeWarning=on
  Unit Delay2 : UnitDelay  SampleTime=-1  HasFrameUpgradeWarning=on
  Output : Outport  VectorParamsAs1DForOutWhenUnconnected=off
  wires:
  TimeCount/1 -> CycleTrigger/2(In2)
  Condition/1 -> Switch3/2
  CycleTrigger/1(Trigger) -> Switch2/2, Unit Delay1/1
  Constant8/1 -> Switch2/1
  Constant10/1 -> Switch2/3
  Switch3/1 -> CycleTrigger/1(In1)
  Constant11/1 -> Switch3/3
  Unit Delay2/1 -> Switch3/1
  Switch2/1 -> Unit Delay2/1
  Unit Delay1/1 -> Output/1

== system EPT/Foreground_TimeBase_5ms/E//W /BP-OBU_E//W/BP-OBU_E//W/BP-OBU_Warning//Fault_G5/Delay41 ==
  Condition : Inport
  TimeCount : Inport  Port=2
  Constant10 : Constant
  Constant11 : Constant  Value=0
  Constant8 : Constant  Value=0
  CycleTrigger : Subsystem
  Switch2 : Switch  Threshold=1
  Switch3 : Switch  Threshold=1
  Unit Delay1 : UnitDelay  SampleTime=-1  HasFrameUpgradeWarning=on
  Unit Delay2 : UnitDelay  SampleTime=-1  HasFrameUpgradeWarning=on
  Output : Outport  VectorParamsAs1DForOutWhenUnconnected=off
  wires:
  Unit Delay1/1 -> Output/1
  Switch2/1 -> Unit Delay2/1
  Unit Delay2/1 -> Switch3/1
  Constant11/1 -> Switch3/3
  Switch3/1 -> CycleTrigger/1(In1)
  Constant10/1 -> Switch2/3
  Constant8/1 -> Switch2/1
  CycleTrigger/1(Trigger) -> Unit Delay1/1, Switch2/2
  Condition/1 -> Switch3/2
  TimeCount/1 -> CycleTrigger/2(In2)

== system EPT/Foreground_TimeBase_5ms/E//W /BP-OBU_E//W/BP-OBU_E//W/BP-OBU_Warning//Fault_G5/Delay42 ==
  Condition : Inport
  TimeCount : Inport  Port=2
  Constant10 : Constant
  Constant11 : Constant  Value=0
  Constant8 : Constant  Value=0
  CycleTrigger : Subsystem
  Switch2 : Switch  Threshold=1
  Switch3 : Switch  Threshold=1
  Unit Delay1 : UnitDelay  SampleTime=-1  HasFrameUpgradeWarning=on
  Unit Delay2 : UnitDelay  SampleTime=-1  HasFrameUpgradeWarning=on
  Output : Outport  VectorParamsAs1DForOutWhenUnconnected=off
  wires:
  TimeCount/1 -> CycleTrigger/2(In2)
  Condition/1 -> Switch3/2
  CycleTrigger/1(Trigger) -> Switch2/2, Unit Delay1/1
  Constant8/1 -> Switch2/1
  Constant10/1 -> Switch2/3
  Switch3/1 -> CycleTrigger/1(In1)
  Constant11/1 -> Switch3/3
  Unit Delay2/1 -> Switch3/1
  Switch2/1 -> Unit Delay2/1
  Unit Delay1/1 -> Output/1

== system EPT/Foreground_TimeBase_5ms/E//W /BP-OBU_E//W/BP-OBU_E//W/BP-OBU_Warning//Fault_G5/Delay43 ==
  Condition : Inport
  TimeCount : Inport  Port=2
  Constant10 : Constant
  Constant11 : Constant  Value=0
  Constant8 : Constant  Value=0
  CycleTrigger : Subsystem
  Switch2 : Switch  Threshold=1
  Switch3 : Switch  Threshold=1
  Unit Delay1 : UnitDelay  SampleTime=-1  HasFrameUpgradeWarning=on
  Unit Delay2 : UnitDelay  SampleTime=-1  HasFrameUpgradeWarning=on
  Output : Outport  VectorParamsAs1DForOutWhenUnconnected=off
  wires:
  Unit Delay1/1 -> Output/1
  Switch2/1 -> Unit Delay2/1
  Unit Delay2/1 -> Switch3/1
  Constant11/1 -> Switch3/3
  Switch3/1 -> CycleTrigger/1(In1)
  Constant10/1 -> Switch2/3
  Constant8/1 -> Switch2/1
  CycleTrigger/1(Trigger) -> Unit Delay1/1, Switch2/2
  Condition/1 -> Switch3/2
  TimeCount/1 -> CycleTrigger/2(In2)

== system EPT/Foreground_TimeBase_5ms/E//W /BP-OBU_E//W/BP-OBU_E//W/BP-OBU_Warning//Fault_G5/Delay44 ==
  Condition : Inport
  TimeCount : Inport  Port=2
  Constant10 : Constant
  Constant11 : Constant  Value=0
  Constant8 : Constant  Value=0
  CycleTrigger : Subsystem
  Switch2 : Switch  Threshold=1
  Switch3 : Switch  Threshold=1
  Unit Delay1 : UnitDelay  SampleTime=-1  HasFrameUpgradeWarning=on
  Unit Delay2 : UnitDelay  SampleTime=-1  HasFrameUpgradeWarning=on
  Output : Outport  VectorParamsAs1DForOutWhenUnconnected=off
  wires:
  TimeCount/1 -> CycleTrigger/2(In2)
  Condition/1 -> Switch3/2
  CycleTrigger/1(Trigger) -> Switch2/2, Unit Delay1/1
  Constant8/1 -> Switch2/1
  Constant10/1 -> Switch2/3
  Switch3/1 -> CycleTrigger/1(In1)
  Constant11/1 -> Switch3/3
  Unit Delay2/1 -> Switch3/1
  Switch2/1 -> Unit Delay2/1
  Unit Delay1/1 -> Output/1

== system EPT/Foreground_TimeBase_5ms/E//W /BP-OBU_E//W/BP-OBU_E//W/BP-OBU_Warning//Fault_G5/Latch42 ==
  Latch : Inport
  Reset : Inport  Port=2
  Switch1 : Switch  Criteria=u2 > Threshold
  Switch3 : Switch  Criteria=u2 > Threshold
  Unit Delay1 : UnitDelay  SampleTime=-1  HasFrameUpgradeWarning=on
  Output : Outport  VectorParamsAs1DForOutWhenUnconnected=off
  wires:
  Switch1/1 -> Switch3/3
  Latch/1 -> Switch1/2, Switch1/1
  Reset/1 -> Switch3/2
  Switch3/1 -> Unit Delay1/1, Output/1
  Unit Delay1/1 -> Switch1/3
